simulink model "svpwm_gen_code"  (R2023a)
settings: Solver=FixedStepDiscrete  StartTime=0.0  StopTime=2  FixedStep=1e-6  RelTol=1e-3
values from neighbouring files (symbols this model uses):
  amplitude_voltage = 12    [PMSM_default.m]
  pair_num = 4    [PMSM_default.m]
  svpwm_period = 1/1000    (= 0.001)    [PMSM_default.m]
  torque_Id_integ_limit = 10.0    (= 10)    [PMSM_default.m]
  torque_Id_out_limit = 100.0    (= 100)    [PMSM_default.m]
  torque_Id_pid_i = 5.0    (= 5)    [PMSM_default.m]
  torque_Id_pid_p = 75.0    (= 75)    [PMSM_default.m]
  torque_Iq_integ_limit = 20.0    (= 20)    [PMSM_default.m]
  torque_Iq_out_limit = 100.0    (= 100)    [PMSM_default.m]
  torque_Iq_pid_d = 0.0    (= 0)    [PMSM_default.m]
  torque_Iq_pid_i = 1.0    (= 1)    [PMSM_default.m]
  torque_Iq_pid_p = 1.0    (= 1)    [PMSM_default.m]
libraries: slpidlib x2
settings Model: Creator=72698  LastModifiedBy=72698

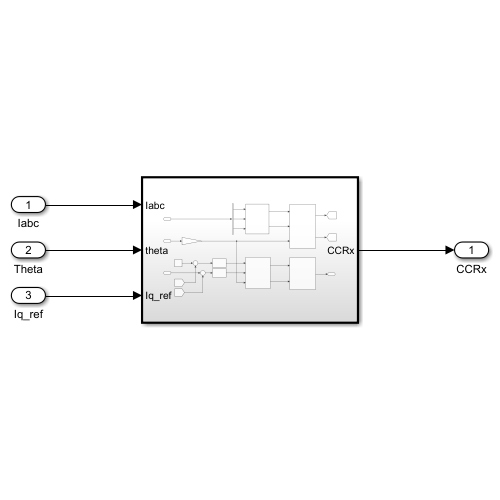
[thumbnail: Simulink's stored preview of the top-level diagram]
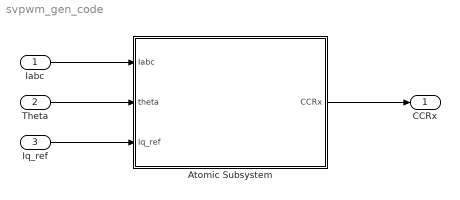
== system svpwm_gen_code ==
  Iabc : Inport
  Theta : Inport  Port=2
  Iq_ref : Inport  Port=3
  Atomic Subsystem : Subsystem  TreatAsAtomicUnit=on
  CCRx : Outport
  wires:
  Iabc/1 -> Atomic Subsystem/1(Iabc)
  Theta/1 -> Atomic Subsystem/2(theta)
  Iq_ref/1 -> Atomic Subsystem/3(Iq_ref)
  Atomic Subsystem/1(CCRx) -> CCRx/1

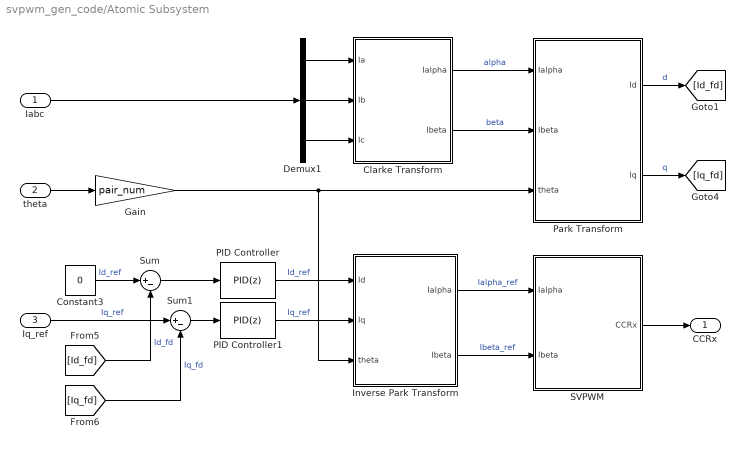
== system svpwm_gen_code/Atomic Subsystem ==
  Iabc : Inport
  theta : Inport  Port=2
  Iq_ref : Inport  Port=3
  Clarke Transform : Subsystem  TreatAsAtomicUnit=on
  Constant3 : Constant  Value=0
  Demux1 : Demux  Outputs=3
  Gain : Gain  Gain=pair_num
  Inverse Park Transform : Subsystem  TreatAsAtomicUnit=on
  PID Controller : slpidlib/PID Controller  Controller=PID  Form=Parallel  TimeDomain=Discrete-time  UseExternalTs=off  SampleTime=-1  IntegratorMethod=Forward Euler  FilterMethod=Forward Euler  ControllerParametersSource=internal  P=torque_Id_pid_p  I=torque_Id_pid_i  UseKiTs=off  D=torque_Iq_pid_d  N=100  UseFilter=on  TunerSelectOption=Transfer Function Based (PID Tuner App)  InitialConditionSource=internal  InitialConditionForIntegrator=0  InitialConditionForFilter=0  DifferentiatorICPrevScaledInput=0  ExternalReset=none  TrackingMode=off  Kt=1  LimitOutput=on  SatLimitsSource=internal  UpperSaturationLimit=torque_Id_out_limit  LowerSaturationLimit=-torque_Id_out_limit  LinearizeAsGain=on  AntiWindupMode=none  Kb=1  LimitIntegrator=on  UpperIntegratorSaturationLimit=torque_Id_integ_limit  LowerIntegratorSaturationLimit=-torque_Id_integ_limit  POutMin=[]  POutMax=[]  IOutMin=[]  IOutMax=[]  DOutMin=[]  DOutMax=[]  NOutMin=[]  NOutMax=[]  SumOutMin=[]  SumOutMax=[]  SaturationOutMin=[]  SaturationOutMax=[]  PParamMin=[]  PParamMax=[]  IParamMin=[]  IParamMax=[]  DParamMin=[]  DParamMax=[]  NParamMin=[]  NParamMax=[]  KbParamMin=[]  KbParamMax=[]  KtParamMin=[]  KtParamMax=[]  KbOutMin=[]  KbOutMax=[]  KtOutMin=[]  KtOutMax=[]  IntegratorOutMin=[]  IntegratorOutMax=[]  FilterOutMin=[]  FilterOutMax=[]  SumI1OutMin=[]  SumI1OutMax=[]  SumI2OutMin=[]  SumI2OutMax=[]  SumI3OutMin=[]  SumI3OutMax=[]  SumI4OutMin=[]  SumI4OutMax=[]  SumDOutMin=[]  SumDOutMax=[]  DifferentiatorOutMin=[]  DifferentiatorOutMax=[]  FilterDiffOutCoefMin=[]  FilterDiffOutCoefMax=[]  ReciprocalOutMin=[]  ReciprocalOutMax=[]  SumDenOutMin=[]  SumDenOutMax=[]  SumNumOutMin=[]  SumNumOutMax=[]  DivideOutMin=[]  DivideOutMax=[]  UdiffTsProdOutMin=[]  UdiffTsProdOutMax=[]  NTsProdOutMin=[]  NTsProdOutMax=[]  UintegralTsProdOutMin=[]  UintegralTsProdOutMax=[]  UngainTsProdOutMin=[]  UngainTsProdOutMax=[]  ClampingZeroOutDataTypeStr=Inherit: Inherit via back propagation  ClampingZeroOutMin=[]  ClampingZeroOutMax=[]  FilterDenConstantOutDataTypeStr=Inherit: Inherit via back propagation  FilterDenConstantOutMin=[]  FilterDenConstantOutMax=[]  PCopyOutDataTypeStr=Inherit: Inherit via back propagation  PCopyOutMin=[]  PCopyOutMax=[]  NCopyOutDataTypeStr=Inherit: Inherit via back propagation  NCopyOutMin=[]  NCopyOutMax=[]  IntegratorContinuousStateAttributes=''  IntegratorStateMustResolveToSignalObject=off  IntegratorRTWStateStorageClass=Auto  FilterContinuousStateAttributes=''  FilterStateMustResolveToSignalObject=off  FilterRTWStateStorageClass=Auto  ParallelPVariant=InternalParameters  IdealPVariant=Disabled  IVariant=InternalParameters  DVariant=InternalParameters  IntegratorVariant=Discrete  SatVariant=Enabled  AWVariant=Passthrough  PCopyVariant=Disabled  TRVariant=Disabled  FdbkBlocksVariant=Forward  IdealPFdbkVariant=Disabled  SatFdbkVariant=Disabled  DerivativeFilterVariant=ForwardEulerFilter  NVariant=InternalParameters  NCopyVariant=Disabled  FilterICVariant=InternalICsFilter  IntegratorICVariant=InternalICs  ExternalResetVariant=Disabled  TRSumVariant=Passthrough  SumFdbkVariant=Disabled  SumVariant=Sum_PID  TsampFilterVariant=InternalTs  TsampNgainVariant=Passthrough  TsampIntegralVariant=Disabled_SignalSpec  ExternalSaturationOutDataTypeStr=Inherit: Same as second input
  PID Controller1 : slpidlib/PID Controller  Controller=PID  Form=Parallel  TimeDomain=Discrete-time  UseExternalTs=off  SampleTime=-1  IntegratorMethod=Forward Euler  FilterMethod=Forward Euler  ControllerParametersSource=internal  P=torque_Iq_pid_p  I=torque_Iq_pid_i  UseKiTs=off  D=torque_Iq_pid_d  N=100  UseFilter=on  TunerSelectOption=Transfer Function Based (PID Tuner App)  InitialConditionSource=internal  InitialConditionForIntegrator=0  InitialConditionForFilter=0  DifferentiatorICPrevScaledInput=0  ExternalReset=none  TrackingMode=off  Kt=1  LimitOutput=on  SatLimitsSource=internal  UpperSaturationLimit=torque_Iq_out_limit  LowerSaturationLimit=-torque_Iq_out_limit  LinearizeAsGain=on  AntiWindupMode=none  Kb=1  LimitIntegrator=on  UpperIntegratorSaturationLimit=torque_Iq_integ_limit  LowerIntegratorSaturationLimit=-torque_Iq_integ_limit  POutMin=[]  POutMax=[]  IOutMin=[]  IOutMax=[]  DOutMin=[]  DOutMax=[]  NOutMin=[]  NOutMax=[]  SumOutMin=[]  SumOutMax=[]  SaturationOutMin=[]  SaturationOutMax=[]  PParamMin=[]  PParamMax=[]  IParamMin=[]  IParamMax=[]  DParamMin=[]  DParamMax=[]  NParamMin=[]  NParamMax=[]  KbParamMin=[]  KbParamMax=[]  KtParamMin=[]  KtParamMax=[]  KbOutMin=[]  KbOutMax=[]  KtOutMin=[]  KtOutMax=[]  IntegratorOutMin=[]  IntegratorOutMax=[]  FilterOutMin=[]  FilterOutMax=[]  SumI1OutMin=[]  SumI1OutMax=[]  SumI2OutMin=[]  SumI2OutMax=[]  SumI3OutMin=[]  SumI3OutMax=[]  SumI4OutMin=[]  SumI4OutMax=[]  SumDOutMin=[]  SumDOutMax=[]  DifferentiatorOutMin=[]  DifferentiatorOutMax=[]  FilterDiffOutCoefMin=[]  FilterDiffOutCoefMax=[]  ReciprocalOutMin=[]  ReciprocalOutMax=[]  SumDenOutMin=[]  SumDenOutMax=[]  SumNumOutMin=[]  SumNumOutMax=[]  DivideOutMin=[]  DivideOutMax=[]  UdiffTsProdOutMin=[]  UdiffTsProdOutMax=[]  NTsProdOutMin=[]  NTsProdOutMax=[]  UintegralTsProdOutMin=[]  UintegralTsProdOutMax=[]  UngainTsProdOutMin=[]  UngainTsProdOutMax=[]  ClampingZeroOutDataTypeStr=Inherit: Inherit via back propagation  ClampingZeroOutMin=[]  ClampingZeroOutMax=[]  FilterDenConstantOutDataTypeStr=Inherit: Inherit via back propagation  FilterDenConstantOutMin=[]  FilterDenConstantOutMax=[]  PCopyOutDataTypeStr=Inherit: Inherit via back propagation  PCopyOutMin=[]  PCopyOutMax=[]  NCopyOutDataTypeStr=Inherit: Inherit via back propagation  NCopyOutMin=[]  NCopyOutMax=[]  IntegratorContinuousStateAttributes=''  IntegratorStateMustResolveToSignalObject=off  IntegratorRTWStateStorageClass=Auto  FilterContinuousStateAttributes=''  FilterStateMustResolveToSignalObject=off  FilterRTWStateStorageClass=Auto  ParallelPVariant=InternalParameters  IdealPVariant=Disabled  IVariant=InternalParameters  DVariant=InternalParameters  IntegratorVariant=Discrete  SatVariant=Enabled  AWVariant=Passthrough  PCopyVariant=Disabled  TRVariant=Disabled  FdbkBlocksVariant=Forward  IdealPFdbkVariant=Disabled  SatFdbkVariant=Disabled  DerivativeFilterVariant=ForwardEulerFilter  NVariant=InternalParameters  NCopyVariant=Disabled  FilterICVariant=InternalICsFilter  IntegratorICVariant=InternalICs  ExternalResetVariant=Disabled  TRSumVariant=Passthrough  SumFdbkVariant=Disabled  SumVariant=Sum_PID  TsampFilterVariant=InternalTs  TsampNgainVariant=Passthrough  TsampIntegralVariant=Disabled_SignalSpec  ExternalSaturationOutDataTypeStr=Inherit: Same as second input
  Park Transform : Subsystem  TreatAsAtomicUnit=on
  SVPWM : Subsystem  TreatAsAtomicUnit=on
  Sum : Sum  Inputs=|+-
  Sum1 : Sum  Inputs=|+-
  CCRx : Outport
  wires:
  Demux1/2 -> Clarke Transform/2(Ib)
  Sum/1 -> PID Controller/1
  Clarke Transform/2(Ibeta) -> Park Transform/2(Ibeta)  "beta"
  PID Controller1/1 -> Inverse Park Transform/2(Iq)  "Iq_ref"
  [Iq_fd] -> Sum1/2  "Iq_fd"
  Iabc/1 -> Demux1/1
  Park Transform/2(Iq) -> [Iq_fd]  "q"
  PID Controller/1 -> Inverse Park Transform/1(Id)  "Id_ref"
  Demux1/3 -> Clarke Transform/3(Ic)
  Gain/1 -> Park Transform/3(theta), Inverse Park Transform/3(theta)
  Inverse Park Transform/1(Ialpha) -> SVPWM/1(Ialpha)  "Ialpha_ref"
  Inverse Park Transform/2(Ibeta) -> SVPWM/2(Ibeta)  "Ibeta_ref"
  SVPWM/1(CCRx) -> CCRx/1
  [Id_fd] -> Sum/2  "Id_fd"
  Constant3/1 -> Sum/1  "Id_ref"
  Park Transform/1(Id) -> [Id_fd]  "d"
  Clarke Transform/1(Ialpha) -> Park Transform/1(Ialpha)  "alpha"
  theta/1 -> Gain/1
  Demux1/1 -> Clarke Transform/1(Ia)
  Iq_ref/1 -> Sum1/1  "Iq_ref"
  Sum1/1 -> PID Controller1/1

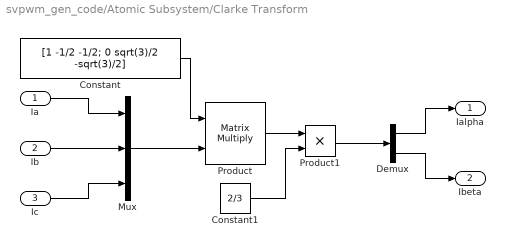
== system svpwm_gen_code/Atomic Subsystem/Clarke Transform ==
  Ia : Inport
  Ib : Inport  Port=2
  Ic : Inport  Port=3
  Constant : Constant  Value=[1 -1/2 -1/2; 0 sqrt(3)/2 -sqrt(3)/2]
  Constant1 : Constant  Value=2/3
  Demux : Demux  Outputs=2
  Mux : Mux  Inputs=3
  Product : Product  Multiplication=Matrix(*)
  Product1 : Product
  Ialpha : Outport
  Ibeta : Outport  Port=2
  wires:
  Ib/1 -> Mux/2
  Ia/1 -> Mux/1
  Ic/1 -> Mux/3
  Mux/1 -> Product/2
  Constant/1 -> Product/1
  Demux/1 -> Ialpha/1
  Demux/2 -> Ibeta/1
  Product/1 -> Product1/1
  Product1/1 -> Demux/1
  Constant1/1 -> Product1/2

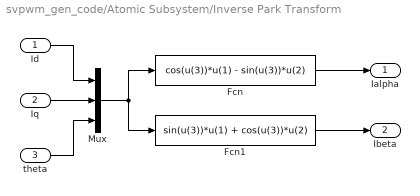
== system svpwm_gen_code/Atomic Subsystem/Inverse Park Transform ==
  Id : Inport
  Iq : Inport  Port=2
  theta : Inport  Port=3
  Fcn : Fcn  Expr=cos(u(3))*u(1) - sin(u(3))*u(2)
  Fcn1 : Fcn  Expr=sin(u(3))*u(1) + cos(u(3))*u(2)
  Mux : Mux  Inputs=3
  Ialpha : Outport
  Ibeta : Outport  Port=2
  wires:
  Iq/1 -> Mux/2
  Id/1 -> Mux/1
  theta/1 -> Mux/3
  Mux/1 -> Fcn/1, Fcn1/1
  Fcn1/1 -> Ibeta/1
  Fcn/1 -> Ialpha/1

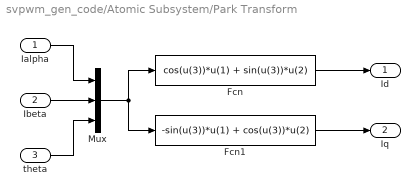
== system svpwm_gen_code/Atomic Subsystem/Park Transform ==
  Ialpha : Inport
  Ibeta : Inport  Port=2
  theta : Inport  Port=3
  Fcn : Fcn  Expr=cos(u(3))*u(1) + sin(u(3))*u(2)
  Fcn1 : Fcn  Expr=-sin(u(3))*u(1) + cos(u(3))*u(2)
  Mux : Mux  Inputs=3
  Id : Outport
  Iq : Outport  Port=2
  wires:
  Ibeta/1 -> Mux/2
  Ialpha/1 -> Mux/1
  theta/1 -> Mux/3
  Mux/1 -> Fcn/1, Fcn1/1
  Fcn1/1 -> Iq/1
  Fcn/1 -> Id/1

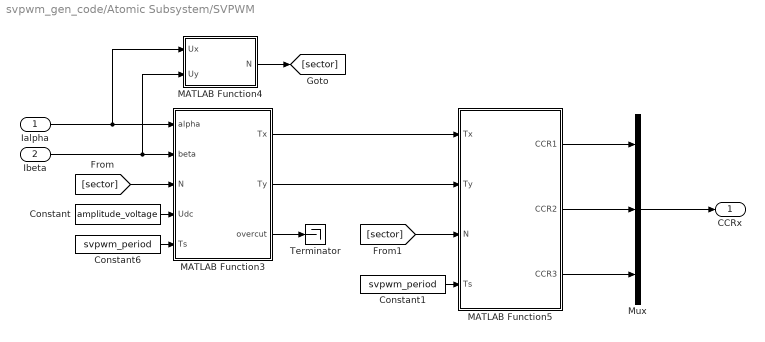
== system svpwm_gen_code/Atomic Subsystem/SVPWM ==
  Ialpha : Inport
  Ibeta : Inport  Port=2
  Constant : Constant  Value=amplitude_voltage
  Constant1 : Constant  Value=svpwm_period
  Constant6 : Constant  Value=svpwm_period
  MATLAB Function3 : MATLAB Function  TreatAsAtomicUnit=on
  MATLAB Function4 : MATLAB Function  TreatAsAtomicUnit=on
  MATLAB Function5 : MATLAB Function  TreatAsAtomicUnit=on
  Mux : Mux  Inputs=3
  Terminator : Terminator
  CCRx : Outport
  wires:
  Ialpha/1 -> MATLAB Function4/1(Ux), MATLAB Function3/1(alpha)
  Ibeta/1 -> MATLAB Function4/2(Uy), MATLAB Function3/2(beta)
  Constant/1 -> MATLAB Function3/4(Udc)
  MATLAB Function3/1(Tx) -> MATLAB Function5/1(Tx)
  MATLAB Function3/2(Ty) -> MATLAB Function5/2(Ty)
  Constant1/1 -> MATLAB Function5/4(Ts)
  MATLAB Function4/1(N) -> [sector]
  [sector] -> MATLAB Function3/3(N)
  Constant6/1 -> MATLAB Function3/5(Ts)
  [sector] -> MATLAB Function5/3(N)
  MATLAB Function3/3(overcut) -> Terminator/1
  Mux/1 -> CCRx/1
  MATLAB Function5/1(CCR1) -> Mux/1
  MATLAB Function5/2(CCR2) -> Mux/2
  MATLAB Function5/3(CCR3) -> Mux/3

== matlab function svpwm_gen_code/Atomic Subsystem/SVPWM/MATLAB Function4 ==
  data: Ux input; N output; Uy input
function N = fcn(Ux, Uy)
% 为了在单片机内快速判断扇区，因此要尽量规避三角函数操作，所以此处使用直线分隔的方式来判断当前扇区
if Uy > 0
    A = 0;
else
    A = 1;
end

if Uy - sqrt(3)*Ux > 0
    B = 0;
else
    B = 1;
end

if Uy + sqrt(3)*Ux > 0
    C = 0;
else
    C = 1;
end

dec = A*4 + B*2 + C;

switch dec
    case 2
        N = 1;
    case 0
        N = 2;
    case 1
        N = 3;
    case 5
        N = 4;
    case 7
        N= 5;
    otherwise
        N = 6;
end

== matlab function svpwm_gen_code/Atomic Subsystem/SVPWM/MATLAB Function3 ==
  data: alpha input; beta input; N input; Tx output; Ty output; Udc input; Ts input; overcut output
function [Tx, Ty, overcut] = fcn(alpha, beta, N, Udc, Ts)
% 我们规定在旋转过程中，逆时针穿过该扇区时遇到的第一个基向量为v1，第二个基向量为v2
% m:调制比sqrt(3)*|Uref|/Udc
% |Uref|*sin(theta):合成矢量在alpha轴上的分量
% |Uref|*cos(theta):合成矢量在beta轴上的分量
value1 = (sqrt(3)/Udc) * Ts * beta;
value2 = (sqrt(3)/Udc) * Ts * (sqrt(3)*alpha + beta)* 0.5;
value3 = (sqrt(3)/Udc) * Ts * (-sqrt(3)*alpha + beta) * 0.5;

switch N
    case 1
        Tx = -value3;
        Ty = value1;
    case 2
        Tx = value3;
        Ty = value2;
    case 3
        Tx = value1;
        Ty = -value2;
    case 4
        Tx = -value1;
        Ty = value3;
    case 5
        Tx = -value2;
        Ty = -value3;
    otherwise
        Tx = value2;
        Ty = -value1;
end

if Tx+Ty > Ts
    overcut = 1;
    Tx_p = Tx; Ty_p = Ty;
    Tx = Ts * Tx_p / (Tx_p+Ty_p);
    Ty = Ts * Ty_p / (Tx_p+Ty_p);
else
    overcut = 0;
end

== matlab function svpwm_gen_code/Atomic Subsystem/SVPWM/MATLAB Function5 ==
  data: Tx input; CCR1 output; Ty input; N input; CCR2 output; CCR3 output; Ts input
function [CCR1, CCR2, CCR3] = fcn(Tx, Ty, N, Ts)

value1 = (Ts-Tx-Ty) / 4;
value2 = value1 + Tx/2;
value3 = value2 + Ty/2;

switch N
    case 1
        CCR1 = value1;
        CCR2 = value2;
        CCR3 = value3;
    case 2
        CCR1 = value2;
        CCR2 = value1;
        CCR3 = value3;
    case 3
        CCR1 = value3;
        CCR2 = value1;
        CCR3 = value2;
    case 4
        CCR1 = value3;
        CCR2 = value2;
        CCR3 = value1;
    case 5
        CCR1 = value2;
        CCR2 = value3;
        CCR3 = value1;
    otherwise
        CCR1 = value1;
        CCR2 = value3;
        CCR3 = value2;
end
